simulink model "Robotic_leg_1"  (R2019b)
settings: Solver=VariableStepAuto  StartTime=0.0  StopTime=10.0  RelTol=1e-3
model workspace (MATLAB code in the model file):
  | %%
  | %dimensions in cm.
  | foot_l = 11.7;
  | foot_w = 5;
  | foot_h = 2;
  | support_w = 4;
  | support_l = 2.5;
  | support_h = 5.5;
  | motor_w = 3.3;
  | motor_l = 3;
  | motor_h = 5.4;
  | link_r = 0.6;
  | link1_l = 19.4;
  | link2_l = 15;
  | hip_l = 9;
  | hip_w = 6;
  | hip_h = 4;
  | 
  | %mass and inertia
  | %damping and stiffness
  | surface_damping = 1e2;
  | surface_stiffness = 1e4;
  | 
  | foot_m = 20;
  | support_m = 20;
  | motor_m = 57.2;
  | link_m = 20;
  | hip_m = 30;
  | 
  | %%
  | m = 3.6;%0.3216;
  | g = 9.81;
  | 
  | Zc = 0.35; %0.3825;
  | w = sqrt(g/Zc);
  | 
  | init_velocity = 0.1;
  | X0 = 0;
  | init_CP = X0 + init_velocity/w;
  | 
  | A = [-w w;0 w];
  | B = [0;-w];
  | C = [1 0];
  | 
  | Q = diag([1,1]);
  | R = 1;
  | 
  | G = lqr(A,B,Q,R);
  | 
  | VV = 1;
  | WW = 1;
  | 
  | OG = lqe(A,B,C,VV,WW);
  | %
undefined symbols (not defined in the file or in its folder): X, Y, Z
libraries: sm_lib x38, nesl_utility x9, Contact_Forces_Lib x5
(part 2 of 2)

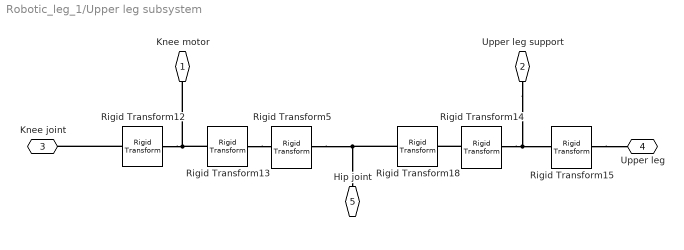
== system Robotic_leg_1/Upper leg subsystem ==
  Rigid Transform12 : sm_lib/Frames and Transforms/Rigid Transform  TranslationMethod=Cartesian  TranslationStandardOffset=0  TranslationLengthUnit=cm  TranslationStandardAxis=+Z  TranslationCartesianOffset=[0 0 -motor_h/2]  TranslationROffset=0  TranslationROffsetUnits=m  TranslationZOffset=0  TranslationZOffsetUnits=m  TranslationThetaOffset=0  TranslationThetaOffsetUnits=deg  RotationMethod=StandardAxis  RotationAngleUnits=deg  RotationStandardAxis=+Y  RotationAngle=90.0  RotationArbitraryAxis=[0 0 1]  FollAlignAxisA=+X  BaseAlignAxisA=+Y  FollAlignAxisB=+Y  BaseAlignAxisB=+Z  RotationSequenceAxes=FollowerAxes  RotationSequence=XYX  RotationSequenceAngles=[0 0 0]  RotationSequenceAnglesUnits=deg  RotationMatrix=[1 0 0; 0 1 0; 0 0 1]
  Rigid Transform13 : sm_lib/Frames and Transforms/Rigid Transform  TranslationMethod=Cartesian  TranslationStandardOffset=0  TranslationLengthUnit=cm  TranslationStandardAxis=+Z  TranslationCartesianOffset=[0 0 motor_h/2]  TranslationROffset=0  TranslationROffsetUnits=m  TranslationZOffset=0  TranslationZOffsetUnits=m  TranslationThetaOffset=0  TranslationThetaOffsetUnits=deg  RotationMethod=None  RotationAngleUnits=deg  RotationStandardAxis=+Z  RotationAngle=0.0  RotationArbitraryAxis=[0 0 1]  FollAlignAxisA=+X  BaseAlignAxisA=+Y  FollAlignAxisB=+Y  BaseAlignAxisB=+Z  RotationSequenceAxes=FollowerAxes  RotationSequence=XYX  RotationSequenceAngles=[0 0 0]  RotationSequenceAnglesUnits=deg  RotationMatrix=[1 0 0; 0 1 0; 0 0 1]
  Rigid Transform14 : sm_lib/Frames and Transforms/Rigid Transform  TranslationMethod=Cartesian  TranslationStandardOffset=0  TranslationLengthUnit=cm  TranslationStandardAxis=+Z  TranslationCartesianOffset=[0 0 -support_h/2]  TranslationROffset=0  TranslationROffsetUnits=m  TranslationZOffset=0  TranslationZOffsetUnits=m  TranslationThetaOffset=0  TranslationThetaOffsetUnits=deg  RotationMethod=None  RotationAngleUnits=deg  RotationStandardAxis=+Z  RotationAngle=0.0  RotationArbitraryAxis=[0 0 1]  FollAlignAxisA=+X  BaseAlignAxisA=+Y  FollAlignAxisB=+Y  BaseAlignAxisB=+Z  RotationSequenceAxes=FollowerAxes  RotationSequence=XYX  RotationSequenceAngles=[0 0 0]  RotationSequenceAnglesUnits=deg  RotationMatrix=[1 0 0; 0 1 0; 0 0 1]
  Rigid Transform15 : sm_lib/Frames and Transforms/Rigid Transform  TranslationMethod=Cartesian  TranslationStandardOffset=0  TranslationLengthUnit=cm  TranslationStandardAxis=+Z  TranslationCartesianOffset=[0 0 support_h/2]  TranslationROffset=0  TranslationROffsetUnits=m  TranslationZOffset=0  TranslationZOffsetUnits=m  TranslationThetaOffset=0  TranslationThetaOffsetUnits=deg  RotationMethod=StandardAxis  RotationAngleUnits=deg  RotationStandardAxis=+Y  RotationAngle=90.0  RotationArbitraryAxis=[0 0 1]  FollAlignAxisA=+X  BaseAlignAxisA=+Y  FollAlignAxisB=+Y  BaseAlignAxisB=+Z  RotationSequenceAxes=FollowerAxes  RotationSequence=XYX  RotationSequenceAngles=[0 0 0]  RotationSequenceAnglesUnits=deg  RotationMatrix=[1 0 0; 0 1 0; 0 0 1]
  Rigid Transform18 : sm_lib/Frames and Transforms/Rigid Transform  TranslationMethod=Cartesian  TranslationStandardOffset=0  TranslationLengthUnit=cm  TranslationStandardAxis=+Z  TranslationCartesianOffset=[0 0 link2_l/2]  TranslationROffset=0  TranslationROffsetUnits=m  TranslationZOffset=0  TranslationZOffsetUnits=m  TranslationThetaOffset=0  TranslationThetaOffsetUnits=deg  RotationMethod=None  RotationAngleUnits=deg  RotationStandardAxis=+Y  RotationAngle=90  RotationArbitraryAxis=[0 0 1]  FollAlignAxisA=+X  BaseAlignAxisA=+Y  FollAlignAxisB=+Y  BaseAlignAxisB=+Z  RotationSequenceAxes=FollowerAxes  RotationSequence=XYX  RotationSequenceAngles=[0 0 0]  RotationSequenceAnglesUnits=deg  RotationMatrix=[1 0 0; 0 1 0; 0 0 1]
  Rigid Transform5 : sm_lib/Frames and Transforms/Rigid Transform  TranslationMethod=Cartesian  TranslationStandardOffset=0  TranslationLengthUnit=cm  TranslationStandardAxis=+Z  TranslationCartesianOffset=[0 0 -link2_l/2]  TranslationROffset=0  TranslationROffsetUnits=m  TranslationZOffset=0  TranslationZOffsetUnits=m  TranslationThetaOffset=0  TranslationThetaOffsetUnits=deg  RotationMethod=None  RotationAngleUnits=deg  RotationStandardAxis=+Y  RotationAngle=90  RotationArbitraryAxis=[0 0 1]  FollAlignAxisA=+X  BaseAlignAxisA=+Y  FollAlignAxisB=+Y  BaseAlignAxisB=+Z  RotationSequenceAxes=FollowerAxes  RotationSequence=XYX  RotationSequenceAngles=[0 0 0]  RotationSequenceAnglesUnits=deg  RotationMatrix=[1 0 0; 0 1 0; 0 0 1]
  Knee motor : PMIOPort  Side=Left
  Upper leg support : PMIOPort  Port=2  Side=Left
  Knee joint : PMIOPort  Port=3  Side=Left
  Upper leg : PMIOPort  Port=4  Side=Right
  Hip joint : PMIOPort  Port=5  Side=Right
  connections:
  Rigid Transform13/RConn1 -- Rigid Transform5/RConn1
  Rigid Transform12/LConn1 -- Rigid Transform13/LConn1 -- Knee motor/RConn1
  Rigid Transform15/RConn1 -- Upper leg/RConn1
  Rigid Transform18/LConn1 -- Rigid Transform5/LConn1 -- Hip joint/RConn1
  Rigid Transform14/LConn1 -- Rigid Transform15/LConn1 -- Upper leg support/RConn1
  Rigid Transform14/RConn1 -- Rigid Transform18/RConn1
  Rigid Transform12/RConn1 -- Knee joint/RConn1

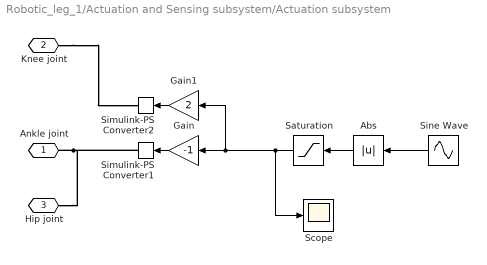
== system Robotic_leg_1/Actuation and Sensing subsystem/Actuation subsystem ==
  Abs : Abs
  Gain : Gain  Gain=-1
  Gain1 : Gain  Gain=2
  Saturation : Saturate  UpperLimit=30  LowerLimit=pi/20
  Scope : Scope
  Simulink-PS Converter1 : nesl_utility/Simulink-PS Converter  PhysicalDomain=network_engine_domain  SubClassName=ps_input  LeftPortType=input  RightPortType=output  PseudoPeriodic=off  Frequencies=[]  NoiseDistribution=none  NoiseParameters=[]  Unit=deg  AffineConversion=off  FilteringAndDerivatives=filter  SimscapeFilterOrder=2  InputFilterTimeConstant=0.01  UdotUserProvided=0
  Simulink-PS Converter2 : nesl_utility/Simulink-PS Converter  PhysicalDomain=network_engine_domain  SubClassName=ps_input  LeftPortType=input  RightPortType=output  PseudoPeriodic=off  Frequencies=[]  NoiseDistribution=none  NoiseParameters=[]  Unit=deg  AffineConversion=off  FilteringAndDerivatives=filter  SimscapeFilterOrder=2  InputFilterTimeConstant=0.01  UdotUserProvided=0
  Sine Wave : Sin  Amplitude=30  Frequency=2*pi/20  Phase=pi/20  Samples=20  SampleTime=0  Offset=1
  Ankle joint : PMIOPort  Side=Right
  Knee joint : PMIOPort  Tag=PMCPort  Port=2  Side=Right
  Hip joint : PMIOPort  Tag=PMCPort  Port=3  Side=Right
  wires:
  Gain/1 -> Simulink-PS Converter1/1
  Sine Wave/1 -> Abs/1
  Abs/1 -> Saturation/1
  Gain1/1 -> Simulink-PS Converter2/1
  Saturation/1 -> Scope/1, Gain1/1, Gain/1
  connections:
  Ankle joint/RConn1 -- Simulink-PS Converter1/RConn1 -- Hip joint/RConn1
  Knee joint/RConn1 -- Simulink-PS Converter2/RConn1

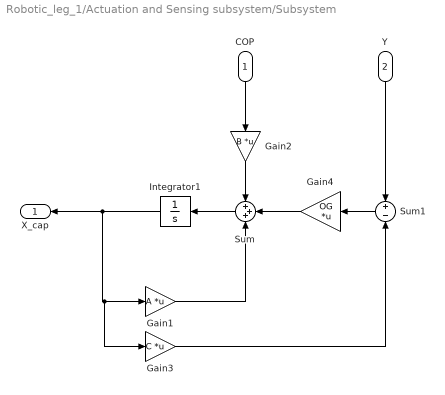
== system Robotic_leg_1/Actuation and Sensing subsystem/Subsystem ==
  COP : Inport
  Y : Inport  Port=2
  Gain1 : Gain  Gain=A  Multiplication=Matrix(K*u)
  Gain2 : Gain  Gain=B  Multiplication=Matrix(K*u)
  Gain3 : Gain  Gain=C  Multiplication=Matrix(K*u)
  Gain4 : Gain  Gain=OG  Multiplication=Matrix(K*u)
  Integrator1 : Integrator  InitialCondition=[0;0]
  Sum : Sum  Inputs=+++
  Sum1 : Sum  Inputs=+|-
  X_cap : Outport
  wires:
  Sum/1 -> Integrator1/1
  Gain3/1 -> Sum1/2
  Gain1/1 -> Sum/3
  COP/1 -> Gain2/1
  Integrator1/1 -> X_cap/1, Gain3/1, Gain1/1
  Gain4/1 -> Sum/2
  Sum1/1 -> Gain4/1
  Gain2/1 -> Sum/1
  Y/1 -> Sum1/1

== matlab function Robotic_leg_1/Actuation and Sensing subsystem/MATLAB Function ==
  data: x input; xdot output; Px input; y output
function [xdot,y] = fcn(x,Px)

%m = 3.6;%0.3216;
g = 9.81;
Zc = 0.35; %0.3825;
w = sqrt(g/Zc);

xdot1 = -w*x(1) + w*x(2);
xdot2 = w*x(2) - w*Px;

xdot = [xdot1;xdot2];
y = x(1);
end
